simulink model "DOB_simulink"  (R2022b)
settings: Solver=VariableStepAuto  StartTime=0.0  StopTime=30  RelTol=1e-3
libraries: simulink x2
settings Model: Creator=USER  LastModifiedBy=USER

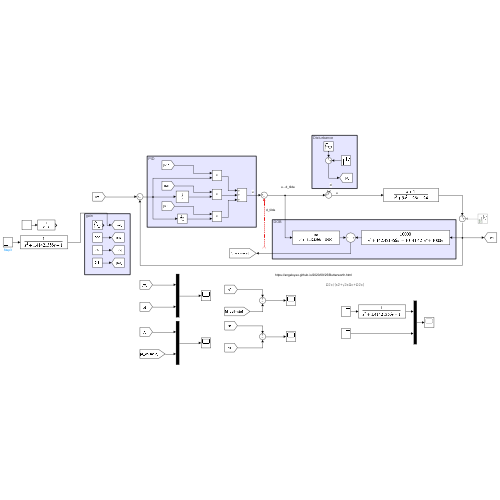
[thumbnail: Simulink's stored preview of the top-level diagram]
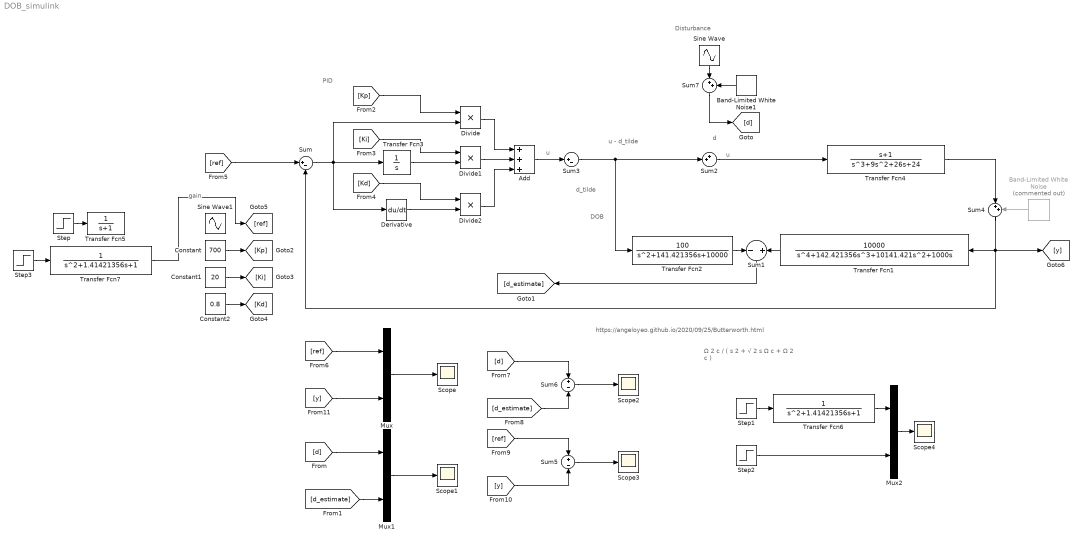
== system DOB_simulink ==
  note: Ω 2 c / ( s 2 + √ 2 s Ω c + Ω 2 c )
  note: https://angeloyeo.github.io/2020/09/25/Butterworth.html
  note: PID
  note: Disturbance
  note: DOB
  note: u - d_tilde
  note: u
  note: gain
  note: d_tilde
  note: d
  note: u
  Add : Sum  Inputs=+++
  Band-Limited White Noise : simulink/Sources/Band-Limited White Noise  Commented=on  Cov=[0.00001]  Ts=0.01  seed=[23341]
  Band-Limited White Noise1 : simulink/Sources/Band-Limited White Noise  Cov=[0.001]  Ts=0.01  seed=[23341]
  Constant : Constant  Value=700
  Constant1 : Constant  Value=20
  Constant2 : Constant  Value=0.8
  Derivative : Derivative
  Divide : Product  Inputs=**
  Divide1 : Product  Inputs=**
  Divide2 : Product  Inputs=**
  Mux : Mux  Inputs=2
  Mux1 : Mux  Inputs=2
  Mux2 : Mux  Inputs=2
  Scope{,1..4} (5 alike) : Scope
  Sine Wave : Sin  Amplitude=20  SampleTime=0
  Sine Wave1 : Sin  Frequency=0.4  SampleTime=0
  Step{,1..3} (4 alike) : Step  SampleTime=0
  Sum : Sum  Inputs=|+-
  Sum1 : Sum  Inputs=-|+
  Sum2 : Sum  Inputs=++|
  Sum3 : Sum  Inputs=|+-
  Sum4 : Sum  Inputs=|++
  Sum5 : Sum  Inputs=+|-
  Sum6 : Sum  Inputs=+|-
  Sum7 : Sum  Inputs=|++
  Transfer Fcn1 : TransferFcn  Numerator=[10000]  Denominator=[1 142.421356 10141.421 1000 0]
  Transfer Fcn2 : TransferFcn  Numerator=[100]  Denominator=[1 141.421356 10000]
  Transfer Fcn3 : TransferFcn  Denominator=[1 0]
  Transfer Fcn4 : TransferFcn  Numerator=[1 1]  Denominator=[1 9 26 24]
  Transfer Fcn5 : TransferFcn  Denominator=[1 1]
  Transfer Fcn6 : TransferFcn  Denominator=[1 1.41421356 1]
  Transfer Fcn7 : TransferFcn  Denominator=[1 1.41421356 1]
  wires:
  [ref] -> Sum/1
  Transfer Fcn2/1 -> Sum1/1
  Sum3/1 -> Sum2/2, Transfer Fcn2/1
  Sum1/1 -> [d_estimate]
  Band-Limited White Noise/1 -> Sum4/2
  Mux/1 -> Scope/1
  [d] -> Mux1/1
  [d_estimate] -> Mux1/2
  Mux1/1 -> Scope1/1
  Add/1 -> Sum3/1
  Sum/1 -> Derivative/1, Transfer Fcn3/1, Divide/2
  Divide1/1 -> Add/2
  Divide2/1 -> Add/3
  [Ki] -> Divide1/1
  [Kp] -> Divide/1
  Transfer Fcn3/1 -> Divide1/2
  Derivative/1 -> Divide2/2
  [Kd] -> Divide2/1
  Divide/1 -> Add/1
  Constant2/1 -> [Kd]
  Constant1/1 -> [Ki]
  Constant/1 -> [Kp]
  [ref] -> Mux/1
  [d_estimate] -> Sum6/2
  [d] -> Sum6/1
  Sum6/1 -> Scope2/1
  Sum5/1 -> Scope3/1
  [ref] -> Sum5/1
  [y] -> Sum5/2
  Sine Wave/1 -> Sum7/1
  Sum7/1 -> [d]
  Band-Limited White Noise1/1 -> Sum7/2
  Sum2/1 -> Transfer Fcn4/1
  Transfer Fcn4/1 -> Sum4/1
  Transfer Fcn1/1 -> Sum1/2
  Sum4/1 -> [y], Sum/2, Transfer Fcn1/1
  [y] -> Mux/2
  ? -> Sum3/2
  Step/1 -> Transfer Fcn5/1
  Step1/1 -> Transfer Fcn6/1
  Transfer Fcn6/1 -> Mux2/1
  Mux2/1 -> Scope4/1
  Step2/1 -> Mux2/2
  Step3/1 -> Transfer Fcn7/1
  Transfer Fcn7/1 -> [ref]
